simulink model "Sem2_Draft1"  (R2018a)
settings: Solver=VariableStepAuto  StartTime=0.0  StopTime=0.0005  RelTol=1e-3
libraries: powerlib x12, simulink x3, powerlib_meascontrol x1
settings Model: Creator=Aditya_Deshmukh  LastModifiedBy=Aditya_Deshmukh
settings SolverCC: ZeroCrossAlgorithm=Adaptive
settings DebuggingCC: MaxConsecutiveZCsMsg=none

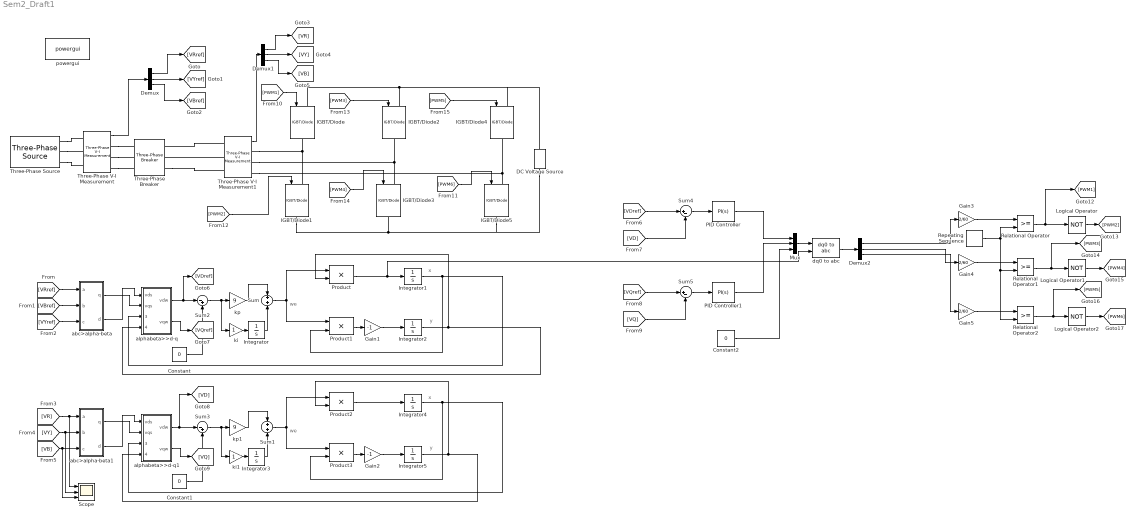
== system Sem2_Draft1 ==
  note: y
  note: x
  note: we
  note: x
  note: y
  note: we
  Constant : Constant  Value=0  VectorParams1D=off
  Constant1 : Constant  Value=0  VectorParams1D=off
  Constant2 : Constant  Value=0
  DC Voltage Source : powerlib/Electrical Sources/DC Voltage Source  Amplitude=600  Measurements=None
  Demux : Demux  Outputs=3
  Demux1 : Demux  Outputs=3
  Demux2 : Demux  Outputs=3
  Gain1 : Gain  Gain=-1  SaturateOnIntegerOverflow=on  OutDataTypeStr=Inherit: Same as input  ParamDataTypeStr=Inherit: Same as input
  Gain2 : Gain  Gain=-1  SaturateOnIntegerOverflow=on  OutDataTypeStr=Inherit: Same as input  ParamDataTypeStr=Inherit: Same as input
  Gain3 : Gain  Gain=2/60
  Gain4 : Gain  Gain=2/60
  Gain5 : Gain  Gain=2/60
  IGBT/Diode{,1..5} (6 alike) : powerlib/Power Electronics/IGBT//Diode  Ron=1e-3  Rs=1e5  Cs=inf  Measurements=off
  Integrator : Integrator
  Integrator1 : Integrator  InitialCondition=1  LimitOutput=on  UpperSaturationLimit=1  LowerSaturationLimit=-1
  Integrator2 : Integrator  LimitOutput=on  UpperSaturationLimit=1  LowerSaturationLimit=-1
  Integrator3 : Integrator
  Integrator4 : Integrator  InitialCondition=1  LimitOutput=on  UpperSaturationLimit=1  LowerSaturationLimit=-1
  Integrator5 : Integrator  LimitOutput=on  UpperSaturationLimit=1  LowerSaturationLimit=-1
  Logical Operator : Logic  Operator=NOT  AllPortsSameDT=off  OutDataTypeStr=boolean
  Logical Operator1 : Logic  Operator=NOT  AllPortsSameDT=off  OutDataTypeStr=boolean
  Logical Operator2 : Logic  Operator=NOT  AllPortsSameDT=off  OutDataTypeStr=boolean
  Mux : Mux  Inputs=3
  PID Controller : simulink/Continuous/PID Controller  Controller=PI  TimeDomain=Continuous-time  SampleTime=-1  IntegratorMethod=Forward Euler  FilterMethod=Forward Euler  Form=Parallel  UseFilter=on  ControllerParametersSource=internal  P=1  I=1  D=0  N=100  InitialConditionSource=internal  InitialConditionForIntegrator=0  InitialConditionForFilter=0  ExternalReset=none  LimitOutput=off  UpperSaturationLimit=inf  LowerSaturationLimit=-inf  LinearizeAsGain=on  AntiWindupMode=none  Kb=1  TrackingMode=off  Kt=1  PParamMin=[]  PParamMax=[]  IParamMin=[]  IParamMax=[]  DParamMin=[]  DParamMax=[]  NParamMin=[]  NParamMax=[]  KbParamMin=[]  KbParamMax=[]  KtParamMin=[]  KtParamMax=[]  POutMin=[]  POutMax=[]  IOutMin=[]  IOutMax=[]  DOutMin=[]  DOutMax=[]  NOutMin=[]  NOutMax=[]  KbOutMin=[]  KbOutMax=[]  KtOutMin=[]  KtOutMax=[]  IntegratorOutMin=[]  IntegratorOutMax=[]  FilterOutMin=[]  FilterOutMax=[]  SumOutMin=[]  SumOutMax=[]  SumI1OutMin=[]  SumI1OutMax=[]  SumI2OutMin=[]  SumI2OutMax=[]  SumI3OutMin=[]  SumI3OutMax=[]  SumDOutMin=[]  SumDOutMax=[]  SaturationOutMin=[]  SaturationOutMax=[]  IntegratorContinuousStateAttributes=''  IntegratorStateMustResolveToSignalObject=off  IntegratorRTWStateStorageClass=Auto  FilterContinuousStateAttributes=''  FilterStateMustResolveToSignalObject=off  FilterRTWStateStorageClass=Auto  DifferentiatorICPrevScaledInput=0  DifferentiatorOutMin=[]  DifferentiatorOutMax=[]  FilterDiffOutCoefMin=[]  FilterDiffOutCoefMax=[]  SumDenOutMin=[]  SumDenOutMax=[]  SumNumOutMin=[]  SumNumOutMax=[]  ReciprocalOutMin=[]  ReciprocalOutMax=[]  DivideOutMin=[]  DivideOutMax=[]  TunerSelectOption=Transfer Function Based (PID Tuner App)
  PID Controller1 : simulink/Continuous/PID Controller  Controller=PI  TimeDomain=Continuous-time  SampleTime=-1  IntegratorMethod=Forward Euler  FilterMethod=Forward Euler  Form=Parallel  UseFilter=on  ControllerParametersSource=internal  P=1  I=1  D=0  N=100  InitialConditionSource=internal  InitialConditionForIntegrator=0  InitialConditionForFilter=0  ExternalReset=none  LimitOutput=off  UpperSaturationLimit=inf  LowerSaturationLimit=-inf  LinearizeAsGain=on  AntiWindupMode=none  Kb=1  TrackingMode=off  Kt=1  PParamMin=[]  PParamMax=[]  IParamMin=[]  IParamMax=[]  DParamMin=[]  DParamMax=[]  NParamMin=[]  NParamMax=[]  KbParamMin=[]  KbParamMax=[]  KtParamMin=[]  KtParamMax=[]  POutMin=[]  POutMax=[]  IOutMin=[]  IOutMax=[]  DOutMin=[]  DOutMax=[]  NOutMin=[]  NOutMax=[]  KbOutMin=[]  KbOutMax=[]  KtOutMin=[]  KtOutMax=[]  IntegratorOutMin=[]  IntegratorOutMax=[]  FilterOutMin=[]  FilterOutMax=[]  SumOutMin=[]  SumOutMax=[]  SumI1OutMin=[]  SumI1OutMax=[]  SumI2OutMin=[]  SumI2OutMax=[]  SumI3OutMin=[]  SumI3OutMax=[]  SumDOutMin=[]  SumDOutMax=[]  SaturationOutMin=[]  SaturationOutMax=[]  IntegratorContinuousStateAttributes=''  IntegratorStateMustResolveToSignalObject=off  IntegratorRTWStateStorageClass=Auto  FilterContinuousStateAttributes=''  FilterStateMustResolveToSignalObject=off  FilterRTWStateStorageClass=Auto  DifferentiatorICPrevScaledInput=0  DifferentiatorOutMin=[]  DifferentiatorOutMax=[]  FilterDiffOutCoefMin=[]  FilterDiffOutCoefMax=[]  SumDenOutMin=[]  SumDenOutMax=[]  SumNumOutMin=[]  SumNumOutMax=[]  ReciprocalOutMin=[]  ReciprocalOutMax=[]  DivideOutMin=[]  DivideOutMax=[]  TunerSelectOption=Transfer Function Based (PID Tuner App)
  Product{,1..3} (4 alike) : Product  SaturateOnIntegerOverflow=on  OutDataTypeStr=Inherit: Same as first input
  Relational Operator : RelationalOperator  OutDataTypeStr=boolean  RndMeth=Simplest
  Relational Operator1 : RelationalOperator  OutDataTypeStr=boolean  RndMeth=Simplest
  Relational Operator2 : RelationalOperator  OutDataTypeStr=boolean  RndMeth=Simplest
  Repeating Sequence : simulink/Sources/Repeating Sequence  rep_seq_t=[0 0.00005 0.0001]  rep_seq_y=[-1 1 -1]
  Scope : Scope  NumInputPorts=3
  Sum : Sum  SaturateOnIntegerOverflow=on
  Sum1 : Sum  SaturateOnIntegerOverflow=on
  Sum2 : Sum  Inputs=|-+  SaturateOnIntegerOverflow=on
  Sum3 : Sum  Inputs=|-+  SaturateOnIntegerOverflow=on
  Sum4 : Sum  Inputs=|+-
  Sum5 : Sum  Inputs=|+-
  Three-Phase V-I Measurement : powerlib/Measurements/Three-Phase V-I Measurement  VoltageMeasurement=phase-to-phase  SetLabelV=off  LabelV=Vabc  Vpu=off  VpuLL=off  CurrentMeasurement=no  SetLabelI=off  LabelI=Iabc  Ipu=off  Pbase=100e6  Vbase=500e3  OutputType=Complex  PhasorSimulation=off  PSBequivalent=0
  Three-Phase V-I Measurement1 : powerlib/Measurements/Three-Phase V-I Measurement  VoltageMeasurement=phase-to-phase  SetLabelV=off  LabelV=Vabc  Vpu=off  VpuLL=off  CurrentMeasurement=no  SetLabelI=off  LabelI=Iabc  Ipu=off  Pbase=100e6  Vbase=500e3  OutputType=Complex  PhasorSimulation=off  PSBequivalent=0
  Three-Phase Breaker : powerlib/Elements/Three-Phase Breaker  InitialState=open  SwitchA=on  SwitchB=on  SwitchC=on  SwitchTimes=0.00025  External=off  BreakerResistance=0.01  SnubberResistance=1e6  SnubberCapacitance=inf  Measurements=None
  Three-Phase Source : powerlib/Electrical Sources/Three-Phase Source  InternalConnection=Yg  VoltagePhases=off  Voltage=415  PhaseAngle=0  Voltage_phases=[25e3 25e3 25e3]/sqrt(3)  PhaseAngles_phases=[0 -120 +120]  Frequency=50  NonIdealSource=off  SpecifyImpedance=off  Resistance=0.8929  Inductance=16.58e-3  ShortCircuitLevel=100e6  BaseVoltage=415  XRratio=7  BusType=swing  Pref=10e3  Qref=0  Prefabc=[10e3, 10e3, 10e3]  Qrefabc=[0, 0, 0]  Qmin=-inf  Qmax=inf
  abc>alpha-beta : Subsystem
  abc>alpha-beta1 : Subsystem
  alphabeta>>d-q : Subsystem
  alphabeta>>d-q1 : Subsystem
  dq0 to abc : powerlib_meascontrol/Transformations/dq0 to abc  Alignment=90 degrees behind phase A axis
  ki : Gain  SaturateOnIntegerOverflow=on  OutDataTypeStr=Inherit: Same as input  ParamDataTypeStr=Inherit: Same as input
  ki1 : Gain  SaturateOnIntegerOverflow=on  OutDataTypeStr=Inherit: Same as input  ParamDataTypeStr=Inherit: Same as input
  kp : Gain  Gain=9  SaturateOnIntegerOverflow=on  OutDataTypeStr=Inherit: Same as input  ParamDataTypeStr=Inherit: Same as input
  kp1 : Gain  Gain=9  SaturateOnIntegerOverflow=on  OutDataTypeStr=Inherit: Same as input  ParamDataTypeStr=Inherit: Same as input
  powergui : powerlib/powergui  Priority=1  SimulationMode=Continuous  SampleTime=50e-6  frequency=60  Iterations=50  frequencyindice=50  Pbase=100e6  ErrMax=1e-4  UnitsV=kV  UnitsW=MW  buscounter=0  FunctionMessages=off  echomessages=off  EnableUseOfTLC=off  CurrentSourceSwitches=off  DisableSnubberDevices=off  DisableRonSwitches=off  DisableVfSwitches=off  DisplayEquations=off  SolverType=Tustin/Backward Euler (TBE)  Interpol=off  ExternalGateDelay=off  methode=off  Ts=100  x0status=blocks  SPID=on  SwTol=0  HookPort=off  RestoreLinks=warning  ResistiveCurrentMeasurement=off  Frange=[0:2:500]  Ylog=off  Xlog=on  ShowGrid=off  save=off  variable=ZData  structure=0  ZoomFFT=off  StartTime=0.0  cycles=1  DisplayStyle=1  fundamental=60  FreqAxis=off  MaxFrequency=1000  frequencyindicesteady=1  RmsSteady=1  display=off
  wires:
  Three-Phase V-I Measurement/1 -> Demux/1
  Three-Phase V-I Measurement1/1 -> Demux1/1
  Demux/2 -> [VYref]
  Demux/3 -> [VBref]
  Demux/1 -> [VRref]
  Demux1/2 -> [VY]
  Demux1/3 -> [VB]
  Demux1/1 -> [VR]
  Product/1 -> dq0 to abc/2, Integrator1/1
  abc>alpha-beta/2(d) -> alphabeta>>d-q/1(vds)
  Sum2/1 -> kp/1, ki/1
  ki/1 -> Integrator/1
  Integrator/1 -> Sum/2
  Gain1/1 -> Integrator2/1
  Product1/1 -> Gain1/1
  abc>alpha-beta/1(q) -> alphabeta>>d-q/2(vqs)
  Sum/1 -> Product1/1, Product/1
  Integrator1/1 -> Product1/2, alphabeta>>d-q/3(sin_e)
  Integrator2/1 -> Product/2, alphabeta>>d-q/4(cos_e)
  kp/1 -> Sum/1
  Constant/1 -> Sum2/2
  alphabeta>>d-q/2(vqw) -> [VQref]
  alphabeta>>d-q/1(vdw) -> [VDref], Sum2/1
  [VRref] -> abc>alpha-beta/1(a)
  [VBref] -> abc>alpha-beta/2(b)
  [VYref] -> abc>alpha-beta/3(c)
  alphabeta>>d-q1/1(vdw) -> [VD], Sum3/1
  alphabeta>>d-q1/2(vqw) -> [VQ]
  abc>alpha-beta1/1(q) -> alphabeta>>d-q1/2(vqs)
  Sum1/1 -> Product3/1, Product2/1
  kp1/1 -> Sum1/1
  Sum3/1 -> kp1/1, ki1/1
  Integrator3/1 -> Sum1/2
  Product2/1 -> Integrator4/1
  Product3/1 -> Gain2/1
  ki1/1 -> Integrator3/1
  Integrator5/1 -> Product2/2, alphabeta>>d-q1/4(cos_e)
  Constant1/1 -> Sum3/2
  Gain2/1 -> Integrator5/1
  abc>alpha-beta1/2(d) -> alphabeta>>d-q1/1(vds)
  [VR] -> Scope/1, abc>alpha-beta1/1(a)
  [VY] -> Scope/2, abc>alpha-beta1/2(b)
  [VB] -> Scope/3, abc>alpha-beta1/3(c)
  [VDref] -> Sum4/1
  [VD] -> Sum4/2
  [VQref] -> Sum5/1
  [VQ] -> Sum5/2
  Sum4/1 -> PID Controller/1
  Sum5/1 -> PID Controller1/1
  Integrator4/1 -> Product3/2, alphabeta>>d-q1/3(sin_e)
  PID Controller/1 -> Mux/1
  PID Controller1/1 -> Mux/2
  Constant2/1 -> Mux/3
  Mux/1 -> dq0 to abc/1
  dq0 to abc/1 -> Demux2/1
  Gain4/1 -> Relational Operator1/1
  Gain3/1 -> Relational Operator/1
  Repeating Sequence/1 -> Relational Operator/2, Relational Operator1/2, Relational Operator2/2
  Relational Operator2/1 -> [PWM5], Logical Operator2/1
  Demux2/3 -> Gain5/1
  Relational Operator/1 -> [PWM1], Logical Operator/1
  Demux2/2 -> Gain4/1
  Logical Operator1/1 -> [PWM4]
  Logical Operator2/1 -> [PWM6]
  Demux2/1 -> Gain3/1
  Gain5/1 -> Relational Operator2/1
  Relational Operator1/1 -> [PWM3], Logical Operator1/1
  Logical Operator/1 -> [PWM2]
  [PWM1] -> IGBT/Diode/1
  [PWM6] -> IGBT/Diode5/1
  [PWM2] -> IGBT/Diode1/1
  [PWM3] -> IGBT/Diode2/1
  [PWM4] -> IGBT/Diode3/1
  [PWM5] -> IGBT/Diode4/1
  connections:
  IGBT/Diode1/LConn1 -- Three-Phase V-I Measurement1/RConn1 -- IGBT/Diode/RConn1
  IGBT/Diode3/LConn1 -- Three-Phase V-I Measurement1/RConn2 -- IGBT/Diode2/RConn1
  IGBT/Diode5/LConn1 -- Three-Phase V-I Measurement1/RConn3 -- IGBT/Diode4/RConn1
  IGBT/Diode/LConn1 -- DC Voltage Source/RConn1 -- IGBT/Diode4/LConn1 -- IGBT/Diode2/LConn1
  IGBT/Diode1/RConn1 -- DC Voltage Source/LConn1 -- IGBT/Diode5/RConn1 -- IGBT/Diode3/RConn1
  Three-Phase V-I Measurement/RConn1 -- Three-Phase Breaker/LConn1
  Three-Phase V-I Measurement/RConn2 -- Three-Phase Breaker/LConn2
  Three-Phase V-I Measurement/RConn3 -- Three-Phase Breaker/LConn3
  Three-Phase Source/RConn1 -- Three-Phase V-I Measurement/LConn1
  Three-Phase Source/RConn2 -- Three-Phase V-I Measurement/LConn2
  Three-Phase Source/RConn3 -- Three-Phase V-I Measurement/LConn3
  Three-Phase V-I Measurement1/LConn2 -- Three-Phase Breaker/RConn2
  Three-Phase V-I Measurement1/LConn1 -- Three-Phase Breaker/RConn1
  Three-Phase Breaker/RConn3 -- Three-Phase V-I Measurement1/LConn3

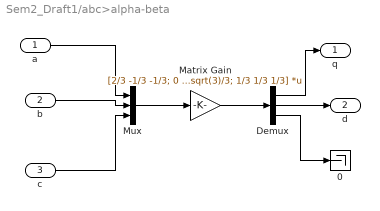
== system Sem2_Draft1/abc>alpha-beta ==
  a : Inport
  b : Inport  Port=2
  c : Inport  Port=3
  0 : Terminator
  Demux : Demux  Outputs=3
  Matrix Gain : Gain  Gain=[2/3 -1/3 -1/3; 0 -sqrt(3)/3 sqrt(3)/3; 1/3 1/3 1/3]  Multiplication=Matrix(K*u)  SaturateOnIntegerOverflow=on  OutDataTypeStr=Inherit: Same as input  ParamDataTypeStr=Inherit: Same as input
  Mux : Mux  Inputs=3
  q : Outport
  d : Outport  Port=2
  wires:
  a/1 -> Mux/1
  b/1 -> Mux/2
  c/1 -> Mux/3
  Demux/1 -> q/1
  Demux/2 -> d/1
  Mux/1 -> Matrix Gain/1
  Matrix Gain/1 -> Demux/1
  Demux/3 -> 0/1

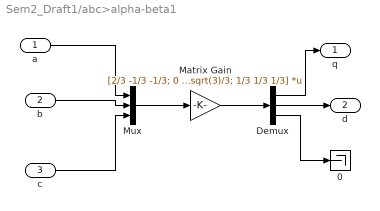
== system Sem2_Draft1/abc>alpha-beta1 ==
  a : Inport
  b : Inport  Port=2
  c : Inport  Port=3
  0 : Terminator
  Demux : Demux  Outputs=3
  Matrix Gain : Gain  Gain=[2/3 -1/3 -1/3; 0 -sqrt(3)/3 sqrt(3)/3; 1/3 1/3 1/3]  Multiplication=Matrix(K*u)  SaturateOnIntegerOverflow=on  OutDataTypeStr=Inherit: Same as input  ParamDataTypeStr=Inherit: Same as input
  Mux : Mux  Inputs=3
  q : Outport
  d : Outport  Port=2
  wires:
  a/1 -> Mux/1
  b/1 -> Mux/2
  c/1 -> Mux/3
  Demux/1 -> q/1
  Demux/2 -> d/1
  Mux/1 -> Matrix Gain/1
  Matrix Gain/1 -> Demux/1
  Demux/3 -> 0/1

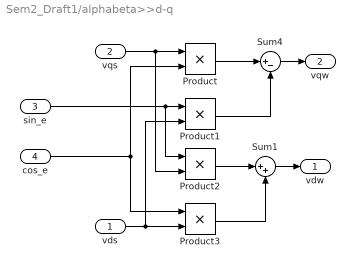
== system Sem2_Draft1/alphabeta>>d-q ==
  vds : Inport
  vqs : Inport  Port=2
  sin_e : Inport  Port=3
  cos_e : Inport  Port=4
  Product{,1..3} (4 alike) : Product  SaturateOnIntegerOverflow=on  RndMeth=Zero  InputSameDT=on  OutDataTypeStr=Inherit: Same as first input
  Sum1 : Sum  Inputs=|++  SaturateOnIntegerOverflow=on  InputSameDT=on  OutDataTypeStr=Inherit: Same as first input
  Sum4 : Sum  Inputs=|+-  SaturateOnIntegerOverflow=on  InputSameDT=on  OutDataTypeStr=Inherit: Same as first input
  vdw : Outport
  vqw : Outport  Port=2
  wires:
  sin_e/1 -> Product1/1, Product2/1
  cos_e/1 -> Product/2, Product3/1
  vqs/1 -> Product2/2, Product/1
  vds/1 -> Product3/2, Product1/2
  Product/1 -> Sum4/1
  Product1/1 -> Sum4/2
  Product2/1 -> Sum1/1
  Product3/1 -> Sum1/2
  Sum4/1 -> vqw/1
  Sum1/1 -> vdw/1

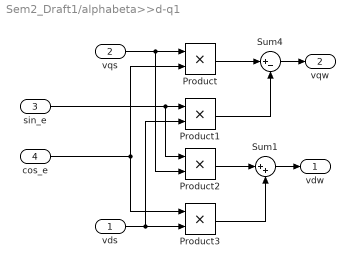
== system Sem2_Draft1/alphabeta>>d-q1 ==
  vds : Inport
  vqs : Inport  Port=2
  sin_e : Inport  Port=3
  cos_e : Inport  Port=4
  Product{,1..3} (4 alike) : Product  SaturateOnIntegerOverflow=on  RndMeth=Zero  InputSameDT=on  OutDataTypeStr=Inherit: Same as first input
  Sum1 : Sum  Inputs=|++  SaturateOnIntegerOverflow=on  InputSameDT=on  OutDataTypeStr=Inherit: Same as first input
  Sum4 : Sum  Inputs=|+-  SaturateOnIntegerOverflow=on  InputSameDT=on  OutDataTypeStr=Inherit: Same as first input
  vdw : Outport
  vqw : Outport  Port=2
  wires:
  sin_e/1 -> Product1/1, Product2/1
  cos_e/1 -> Product/2, Product3/1
  vqs/1 -> Product2/2, Product/1
  vds/1 -> Product3/2, Product1/2
  Product/1 -> Sum4/1
  Product1/1 -> Sum4/2
  Product2/1 -> Sum1/1
  Product3/1 -> Sum1/2
  Sum4/1 -> vqw/1
  Sum1/1 -> vdw/1
